simulink model "CaseDemuxTwo"  (R2023b)
settings: Solver=VariableStepAuto  StartTime=0.0  StopTime=10.0  RelTol=1e-3
settings Model: Creator=jsonm  LastModifiedBy=jsonm

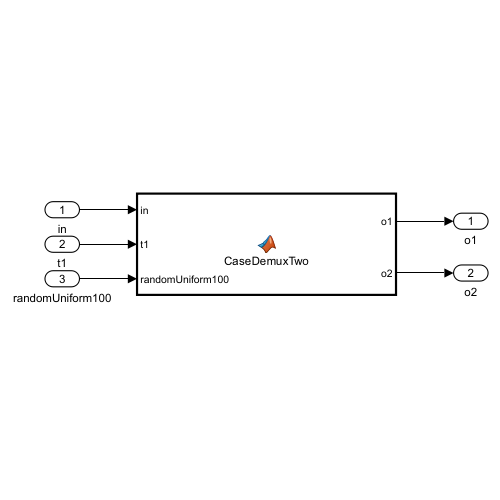
[thumbnail: Simulink's stored preview of the top-level diagram]
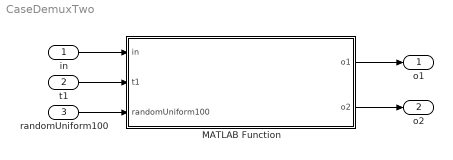
== system CaseDemuxTwo ==
  in : Inport
  t1 : Inport  Port=2
  randomUniform100 : Inport  Port=3
  MATLAB Function : MATLAB Function  TreatAsAtomicUnit=on
  o1 : Outport
  o2 : Outport  Port=2
  wires:
  MATLAB Function/1(o1) -> o1/1
  MATLAB Function/2(o2) -> o2/1
  in/1 -> MATLAB Function/1(in)
  t1/1 -> MATLAB Function/2(t1)
  randomUniform100/1 -> MATLAB Function/3(randomUniform100)

== matlab function CaseDemuxTwo/MATLAB Function ==
  data: in input; o1 output; t1 input; o2 output; randomUniform100 input
function [o1, o2] = CaseDemuxTwo(in, t1, randomUniform100)

% Method to demux input into one of two possible outputs based on
% probabilities.
%
% t1 is a threshold bound between 0 and 100 used as follows
% x = rand*100
% 0 <= x < t1 => o1
%
% Negative is a non-valid output
%
% Written by Darian Muresan
% Modified by Jason McCauley

o1 = -1;
o2 = -1;

if nargin < 3
    x = rand*100; % If randomUniform100 not provided, generate random number inside node
else
    x = randomUniform100; % randomUniform100 uses a different seed to generate each random number, use if provided at each CaseDemux
end

if (0 <= x && x <= t1)
    o1 = in;
else
    o2 = in;
end
